simulink model "sampleModel1848"  (R2023a)
settings: Solver=VariableStepAuto  StartTime=0.0  StopTime=10.0  RelTol=1e-3
libraries: hdlsllib x7, simulink x1
settings Model: Creator=user1  LastModifiedBy=user1

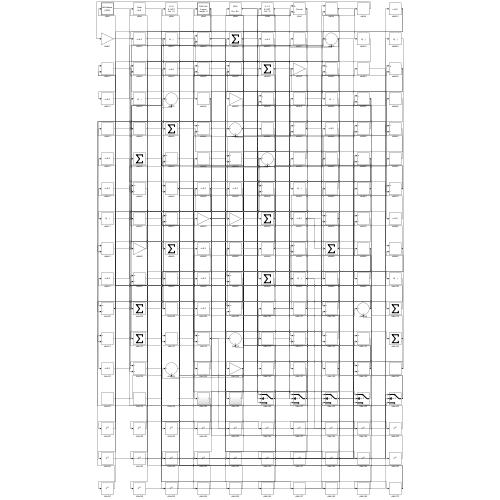
[thumbnail: Simulink's stored preview of the top-level diagram]
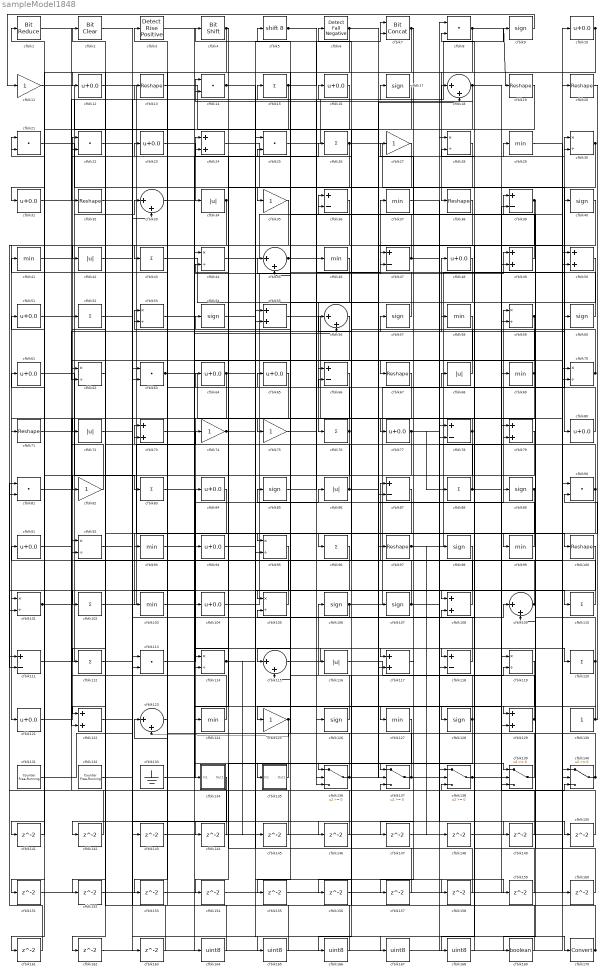
== system sampleModel1848 ==
  cfblk1 : hdlsllib/Logic and Bit Operations/Bit Reduce  mode=AND
  cfblk{10,12,16,23,31,48,51,61,64..65,77,80,84,91,94,104,121} (17 alike) : Bias  Bias=0.0  SaturateOnIntegerOverflow=off
  cfblk{13,19..20,32,38,67,71,97,100} (9 alike) : Reshape
  cfblk{28,30,44,53,59,62,70,92,95,101,105,114,119} (13 alike) : Product  Inputs=*/  RndMeth=Zero  SaturateOnIntegerOverflow=on
  cfblk{15,26,43,52,76,83,88,96,102,110,112,120} (12 alike) : Sum  Inputs=+
  cfblk{29,37,41,46,58,69,93,99,103,124,127} (11 alike) : MinMax
  cfblk{9,17,40,54,57,60,85,89,98,106..107,126,128} (13 alike) : Signum
  cfblk{24,49..50,55,73,79,108,117,122,129} (10 alike) : Sum
  cfblk{18,33,45,56,109,115,123} (7 alike) : Sum  Inputs=|++
  cfblk{11,27,35,74..75,82,125} (7 alike) : Gain
  cfblk{36,39,47,66,78,87,111,118} (8 alike) : Sum  Inputs=+-
  cfblk{8,14,21..22,25,63,81,90,113} (9 alike) : DotProduct  OutDataTypeStr=Inherit: Inherit via internal rule
  cfblk{34,42,68,72,86,116} (6 alike) : Abs  SaturateOnIntegerOverflow=off
  cfblk130 : Constant  SampleTime=-1
  cfblk131 : hdlsllib/Sources/Counter Free-Running  NumBits=16  tsamp=-1
  cfblk132 : hdlsllib/Sources/Counter Free-Running  NumBits=16  tsamp=-1
  cfblk133 : Ground
  cfblk134 : Subsystem
      settings: LibrarySourceBlock=|
      | hdlsllib/Ports &
      | Subsystems/Subsystem
  cfblk135 : Subsystem
      settings: LibrarySourceBlock=|
      | hdlsllib/Ports &
      | Subsystems/Subsystem
  cfblk{136..140} (5 alike) : Switch  SaturateOnIntegerOverflow=off  InputSameDT=off
  cfblk{141..163} (23 alike) : Delay  SampleTime=1
  cfblk{164..168} (5 alike) : DataTypeConversion  OutDataTypeStr=uint8  SaturateOnIntegerOverflow=off  RndMeth=Floor
  cfblk169 : DataTypeConversion  OutDataTypeStr=boolean  SaturateOnIntegerOverflow=off  RndMeth=Floor
  cfblk170 : DataTypeConversion  SaturateOnIntegerOverflow=off  RndMeth=Floor
  cfblk2 : simulink/Logic and Bit Operations/Bit Clear  iBit=0
      settings: LibrarySourceBlock=|
      | hdlsllib/Logic and Bit
      | Operations/Bit Clear
  cfblk3 : hdlsllib/Logic and Bit Operations/Detect Rise Positive  vinit=0  OutDataTypeStr=boolean
  cfblk4 : hdlsllib/Logic and Bit Operations/Bit Shift  mode=Shift Left Logical  N=0
  cfblk5 : ArithShift  BitShiftNumber=8
  cfblk6 : hdlsllib/Logic and Bit Operations/Detect Fall Negative  vinit=0  OutDataTypeStr=boolean
  cfblk7 : hdlsllib/Logic and Bit Operations/Bit Concat  numInputs=2
  wires:
  cfblk60/1 -> cfblk37/1
  cfblk66/1 -> cfblk134/1(In1)
  cfblk34/1 -> cfblk121/1, cfblk113/2
  cfblk10/1 -> cfblk38/1, cfblk43/1
  cfblk8/1 -> cfblk19/1, cfblk63/2
  cfblk2/1 -> cfblk170/1
  cfblk68/1 -> cfblk6/1
  cfblk23/1 -> cfblk34/1
  cfblk69/1 -> cfblk48/1, cfblk135/1(In1)
  cfblk20/1 -> cfblk99/1
  cfblk104/1 -> cfblk49/1
  cfblk50/1 -> cfblk76/1
  cfblk26/1 -> cfblk80/1, cfblk136/3
  cfblk75/1 -> cfblk47/1
  cfblk85/1 -> cfblk46/1
  cfblk5/1 -> cfblk137/1, cfblk128/1
  cfblk96/1 -> cfblk105/1
  cfblk99/1 -> cfblk59/1
  cfblk12/1 -> cfblk100/1
  cfblk138/1 -> cfblk79/1, cfblk140/3
  cfblk101/1 -> cfblk33/1, cfblk21/2
  cfblk126/1 -> cfblk4/1
  cfblk59/1 -> cfblk67/1, cfblk114/2
  cfblk67/1 -> cfblk71/1
  cfblk132/1 -> cfblk33/2
  cfblk120/1 -> cfblk85/1, cfblk139/3
  cfblk71/1 -> cfblk15/1
  cfblk113/1 -> cfblk84/1
  cfblk49/1 -> cfblk27/1
  cfblk124/1 -> cfblk22/1
  cfblk6/1 -> cfblk35/1, cfblk50/2
  cfblk102/1 -> cfblk74/1
  cfblk14/1 -> cfblk117/1, cfblk167/1
  cfblk55/1 -> cfblk90/1
  cfblk97/1 -> cfblk30/1, cfblk148/1
  cfblk4/1 -> cfblk124/1, cfblk31/1, cfblk42/1
  cfblk78/1 -> cfblk137/2, cfblk77/1
  cfblk82/1 -> cfblk32/1
  cfblk44/1 -> cfblk20/1
  cfblk117/1 -> cfblk137/3
  cfblk73/1 -> cfblk57/1
  cfblk87/1 -> cfblk103/1
  cfblk106/1 -> cfblk40/1, cfblk105/2, cfblk89/1
  cfblk81/1 -> cfblk16/1
  cfblk110/1 -> cfblk87/1
  cfblk115/1 -> cfblk118/1
  cfblk21/1 -> cfblk97/1
  cfblk108/1 -> cfblk51/1
  cfblk137/1 -> cfblk65/1, cfblk149/1
  cfblk130/1 -> cfblk129/1, cfblk90/2
  cfblk114/1 -> cfblk145/1, cfblk146/1
  cfblk77/1 -> cfblk88/1, cfblk79/2, cfblk161/1
  cfblk25/1 -> cfblk9/1
  cfblk37/1 -> cfblk78/1
  cfblk129/1 -> cfblk106/1, cfblk53/1
  cfblk45/1 -> cfblk120/1, cfblk18/1
  cfblk31/1 -> cfblk13/1
  cfblk105/1 -> cfblk61/1
  cfblk17/1 -> cfblk93/1
  cfblk98/1 -> cfblk111/2
  cfblk24/1 -> cfblk126/1
  cfblk46/1 -> cfblk95/1
  cfblk116/1 -> cfblk119/2
  cfblk125/1 -> cfblk123/2, cfblk45/2
  cfblk11/1 -> cfblk44/1
  cfblk63/1 -> cfblk98/1, cfblk129/2
  cfblk30/1 -> cfblk114/1, cfblk147/1
  cfblk121/1 -> cfblk92/1
  cfblk133/1 -> cfblk47/2
  cfblk94/1 -> cfblk60/1
  cfblk58/1 -> cfblk75/1
  cfblk79/1 -> cfblk82/1
  cfblk140/1 -> cfblk39/1, cfblk91/1
  cfblk89/1 -> cfblk95/2, cfblk115/1
  cfblk41/1 -> cfblk17/1
  cfblk128/1 -> cfblk54/1, cfblk154/1
  cfblk111/1 -> cfblk10/1
  cfblk70/1 -> cfblk8/2, cfblk22/2
  cfblk136/1 -> cfblk24/1, cfblk30/2
  cfblk27/1 -> cfblk55/2
  cfblk43/1 -> cfblk107/1
  cfblk86/1 -> cfblk64/1, cfblk18/2
  cfblk118/1 -> cfblk5/1
  cfblk54/1 -> cfblk110/1
  cfblk123/1 -> cfblk73/1
  cfblk65/1 -> cfblk101/1
  cfblk56/1 -> cfblk66/1
  cfblk119/1 -> cfblk125/1
  cfblk39/1 -> cfblk36/2, cfblk168/1, cfblk169/1
  cfblk53/1 -> cfblk118/2
  cfblk107/1 -> cfblk78/2, cfblk36/1
  cfblk74/1 -> cfblk139/1, cfblk158/1, cfblk159/1
  cfblk13/1 -> cfblk117/2
  cfblk61/1 -> cfblk83/1
  cfblk92/1 -> cfblk104/1
  cfblk135/1(Out1) -> cfblk41/1
  cfblk38/1 -> cfblk81/2
  cfblk139/1 -> cfblk68/1
  cfblk51/1 -> cfblk62/2
  cfblk40/1 -> cfblk87/2
  cfblk103/1 -> cfblk136/1
  cfblk83/1 -> cfblk26/1
  cfblk16/1 -> cfblk122/1
  cfblk88/1 -> cfblk69/1, cfblk52/1
  cfblk80/1 -> cfblk66/2
  cfblk122/1 -> cfblk109/1
  cfblk48/1 -> cfblk136/2
  cfblk91/1 -> cfblk58/1
  cfblk90/1 -> cfblk56/1, cfblk138/2
  cfblk35/1 -> cfblk101/2
  cfblk64/1 -> cfblk122/2, cfblk7/2, cfblk162/1
  cfblk131/1 -> cfblk94/1
  cfblk62/1 -> cfblk112/1
  cfblk76/1 -> cfblk72/1, cfblk53/2, cfblk153/1
  cfblk57/1 -> cfblk24/2
  cfblk1/1 -> cfblk70/2
  cfblk47/1 -> cfblk25/2, cfblk29/1
  cfblk18/1 -> cfblk139/2, cfblk96/1, cfblk14/2, cfblk115/2
  cfblk33/1 -> cfblk56/2
  cfblk109/1 -> cfblk108/1, cfblk45/1, cfblk21/1
  cfblk9/1 -> cfblk11/1
  cfblk7/1 -> cfblk127/1, cfblk12/1
  cfblk93/1 -> cfblk86/1
  cfblk72/1 -> cfblk14/1
  cfblk15/1 -> cfblk7/1, cfblk102/1
  cfblk19/1 -> cfblk141/1
  cfblk141/1 -> cfblk1/1
  cfblk134/1(Out1) -> cfblk142/1
  cfblk142/1 -> cfblk62/1
  cfblk32/1 -> cfblk143/1
  cfblk143/1 -> cfblk138/1
  cfblk22/1 -> cfblk144/1
  cfblk144/1 -> cfblk92/2
  cfblk145/1 -> cfblk81/1
  cfblk146/1 -> cfblk73/2
  cfblk147/1 -> cfblk140/2
  cfblk148/1 -> cfblk39/2
  cfblk149/1 -> cfblk108/2
  cfblk42/1 -> cfblk150/1
  cfblk150/1 -> cfblk55/1
  cfblk95/1 -> cfblk151/1
  cfblk151/1 -> cfblk119/1
  cfblk84/1 -> cfblk152/1
  cfblk152/1 -> cfblk49/2
  cfblk153/1 -> cfblk140/1
  cfblk154/1 -> cfblk50/1
  cfblk36/1 -> cfblk155/1
  cfblk155/1 -> cfblk8/1
  cfblk127/1 -> cfblk156/1
  cfblk156/1 -> cfblk59/2
  cfblk100/1 -> cfblk157/1
  cfblk157/1 -> cfblk25/1
  cfblk158/1 -> cfblk44/2
  cfblk159/1 -> cfblk138/3
  cfblk29/1 -> cfblk160/1
  cfblk160/1 -> cfblk109/2
  cfblk161/1 -> cfblk111/1
  cfblk162/1 -> cfblk70/1
  cfblk52/1 -> cfblk163/1
  cfblk163/1 -> cfblk63/1
  cfblk3/1 -> cfblk164/1
  cfblk164/1 -> cfblk23/1
  cfblk112/1 -> cfblk165/1
  cfblk165/1 -> cfblk3/1
  cfblk28/1 -> cfblk166/1
  cfblk166/1 -> cfblk113/1
  cfblk167/1 -> cfblk28/1
  cfblk168/1 -> cfblk28/2
  cfblk169/1 -> cfblk2/1
  cfblk170/1 -> cfblk116/1, cfblk123/1

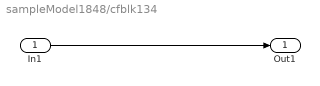
== system sampleModel1848/cfblk134 ==
  In1 : Inport
  Out1 : Outport
  wires:
  In1/1 -> Out1/1

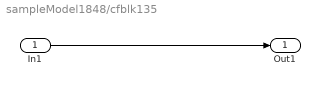
== system sampleModel1848/cfblk135 ==
  In1 : Inport
  Out1 : Outport
  wires:
  In1/1 -> Out1/1
